simulink model "ein_seiten2"  (Simulink 6.1)
settings: Solver=ode45  StartTime=0.0  StopTime=10.0  RelTol=1e-3
values from neighbouring files (symbols this model uses):
  f1 = 0.1    [CFIR_1.m]    (also in analog_bp1.m = ',num2str(f1),' Hz; analog_bp11.m = ',num2str(f1),' Hz; analog_bp2.m = 30000; analog_bp3.m = 30000)
  f2 = 0.3    [CFIR_1.m]    (also in analog_bp1.m = ',num2str(f2),' Hz)']); analog_bp11.m = ',num2str(f2),' Hz)']); analog_bp2.m = 35000; analog_bp3.m = 30500)
  fs = 16000    [G722_1.m]    (also in TP_fdesign1.m = 0.215; adaptiv_2.m = 1000; adaptiv_3.m = 1000; adaptiv_4.m = 1000)
  nord = 6    [analog_bp1.m]    (also in analog_bp2.m; analog_bp3.m; analog_tp1.m = 8; analog_tp2.m = 8)
undefined symbols (not defined in the file or in its folder): b_pm, bc_i, bc_r, get
libraries: dspsnks4 x2, dsparch4 x1, dspbuff3 x1, dspobslib x1, simulink x1, dspspect3 x1, dspsigops x1
settings Model: Creator=svenhoffmann  LastModifiedBy=svenhoffmann  ExtModeAutoUpdateStatusClock=off
settings DataIOCC: MaxDataPoints=1  SignalLoggingName=sigsOut
settings HardwareCC: TargetUnknown=on

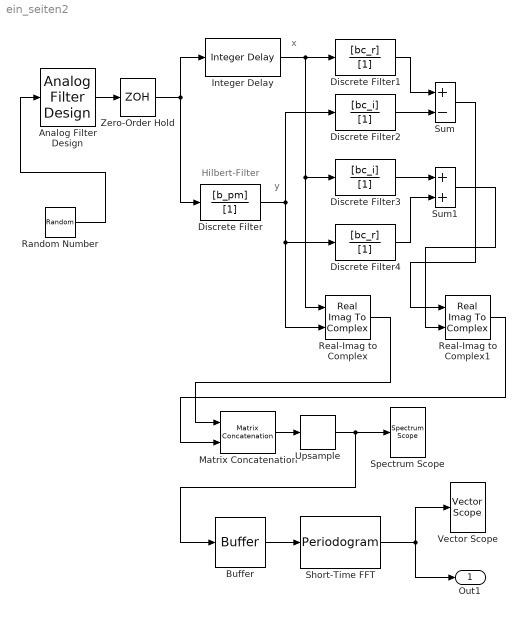
== system ein_seiten2 ==
  note: Hilbert-Filter
  note: x
  note: y
  Analog Filter Design : dsparch4/Analog Filter Design  method=Chebyshev I  filttype=Bandpass  N=8  Wlo=2*pi*f1  Whi=2*pi*f2  Rp=2  Rs=40
  Buffer : dspbuff3/Buffer  N=256  V=64  ic=0
  Discrete Filter : DiscreteFilter  Numerator=[b_pm]  Denominator=[1]  SampleTime=1/fs
  Discrete Filter1 : DiscreteFilter  Numerator=[bc_r]  Denominator=[1]  SampleTime=1/fs
  Discrete Filter2 : DiscreteFilter  Numerator=[bc_i]  Denominator=[1]  SampleTime=1/fs
  Discrete Filter3 : DiscreteFilter  Numerator=[bc_i]  Denominator=[1]  SampleTime=1/fs
  Discrete Filter4 : DiscreteFilter  Numerator=[bc_r]  Denominator=[1]  SampleTime=1/fs
  Integer Delay : dspobslib/Integer Delay  delay=nord/2  ic=0  reset_popup=None
  Matrix Concatenation : simulink/Math Operations/Matrix Concatenation  numInports=2  catMethod=Horizontal
  Random Number : RandomNumber  SampleTime=0
  Real-Imag to Complex : RealImagToComplex
  Real-Imag to Complex1 : RealImagToComplex
  Short-Time FFT : dspspect3/Periodogram  wintype=Hann  Rs=50  beta=5  winsamp=Periodic  inheritFFT=off  fftsize=256  navg=10
  Spectrum Scope : dspsnks4/Spectrum Scope  ScopeProperties=off  Domain=Frequency  HorizSpan=1  UseBuffer=on  BufferSize=256  Overlap=64  inpFftLenInherit=on  FFTlength=256  numAvg=20  DisplayProperties=on  AxisGrid=on  Memory=off  FrameNumber=on  AxisLegend=off  AxisZoom=off  OpenScopeAtSimStart=on  OpenScopeImmediately=off  FigPos=get(0,'defaultfigureposition')  AxisProperties=off  XUnits=Hertz  XRange=[0...Fs]  InheritXIncr=on  XIncr=1.0  XLabel=Samples  YUnits=dB  YLabel=Magnitude, dB  LineProperties=off  wintypeSpecScope=Hann  RsSpecScope=50  betaSpecScope=5  winsampSpecScope=Periodic
      settings: YMin=-164.362377632534  YMax=15.8101220793404
  Sum : Sum  Inputs=+-  SaturateOnIntegerOverflow=on
  Sum1 : Sum  SaturateOnIntegerOverflow=on
  Upsample : dspsigops/Upsample  N=2  phase=0  ic=0  mode=Maintain input frame size
  Vector Scope : dspsnks4/Vector Scope  ScopeProperties=off  Domain=Frequency  HorizSpan=1  DisplayProperties=off  AxisGrid=on  Memory=off  FrameNumber=on  AxisLegend=off  AxisZoom=off  OpenScopeAtSimStart=on  OpenScopeImmediately=off  FigPos=get(0,'defaultfigureposition')  AxisProperties=on  XUnits=Hertz  XRange=[0...Fs]  InheritXIncr=on  XIncr=1/(2*fs)  XLabel=Time  YUnits=dB  YLabel=Amplitude  LineProperties=off
      settings: YMin=-164.362377632534  YMax=15.8101220793404
  Zero-Order Hold : ZeroOrderHold  SampleTime=1/fs
  Out1 : Outport
  wires:
  Analog Filter Design/1 -> Zero-Order Hold/1
  Zero-Order Hold/1 -> Integer Delay/1, Discrete Filter/1
  Integer Delay/1 -> Discrete Filter1/1, Real-Imag to Complex/1, Discrete Filter3/1
  Discrete Filter/1 -> Discrete Filter4/1, Real-Imag to Complex/2, Discrete Filter2/1
  Random Number/1 -> Analog Filter Design/1
  Matrix Concatenation/1 -> Upsample/1
  Buffer/1 -> Short-Time FFT/1
  Short-Time FFT/1 -> Out1/1, Vector Scope/1
  Upsample/1 -> Spectrum Scope/1, Buffer/1
  Discrete Filter2/1 -> Sum/2
  Discrete Filter1/1 -> Sum/1
  Discrete Filter3/1 -> Sum1/1
  Discrete Filter4/1 -> Sum1/2
  Real-Imag to Complex/1 -> Matrix Concatenation/1
  Sum/1 -> Real-Imag to Complex1/1
  Sum1/1 -> Real-Imag to Complex1/2
  Real-Imag to Complex1/1 -> Matrix Concatenation/2
